simulink model "Sim1"  (R2014a)
settings: Solver=ode45  StartTime=0.0  StopTime=10.0  RelTol=1e-3
settings Model: Creator=OCAC  LastModifiedBy=OCAC

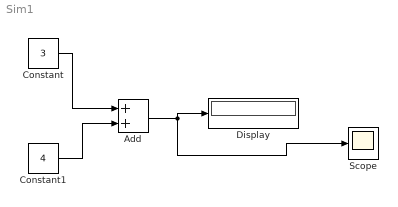
== system Sim1 ==
  Add : Sum
  Constant : Constant  Value=3
  Constant1 : Constant  Value=4
  Display : Display
  Scope : Scope
  wires:
  Constant/1 -> Add/1
  Constant1/1 -> Add/2
  Add/1 -> Display/1, Scope/1
